simulink model "CruiseControl_TestHarness"  (R2020a)
settings: configuration reference "ModelReferencingVisual" (kept outside this file)
libraries: SignalEditorBlockLib x1
settings Model: DataDictionary=CruiseControl_Req_dd.sldd  Creator=colosky  LastModifiedBy=promero
settings ConfigSetRef: SourceName=ModelReferencingVisual

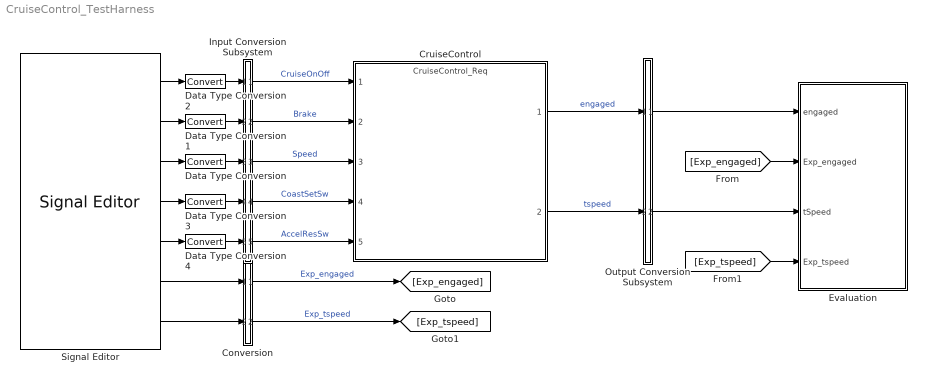
== system CruiseControl_TestHarness ==
  Conversion : Subsystem
      mask Display: disp('');
  CruiseControl : ModelReference  ModelNameDialog=CruiseControl_Req  SimulationMode=Normal  CodeInterface=Top model  ModelReferenceVersion=1.469
  Data Type Conversion{,1..4} (5 alike) : DataTypeConversion
  Evaluation : Subsystem
  Input Conversion Subsystem : Subsystem  Tag=__SLT_ICS__  Description=|
      | Signal spec.
      | and routing
      settings: AttributesFormatString=%<Description>
  Output Conversion Subsystem : Subsystem  Tag=__SLT_OCS__  Description=|
      | Signal spec.
      | and routing
      settings: AttributesFormatString=%<Description>
  Signal Editor : SignalEditorBlockLib/Signal Editor  FileName=TestInputs.mat  ActiveScenario=Engage_AccelResSw_Veh_Spd  ActiveSignal=Speed  IsBus=off  OutputBusObjectStr=Bus: BusObject  SampleTime=0.1  OutputAfterFinalValue=Extrapolation  Unit=inherit  PreserveSignalName=on
  wires:
  Conversion/1(Out6) -> [Exp_engaged]  "Exp_engaged"
  Conversion/2(Out7) -> [Exp_tspeed]  "Exp_tspeed"
  Output Conversion Subsystem/1(Outport_1) -> Evaluation/1(engaged)
  Output Conversion Subsystem/2(Outport_2) -> Evaluation/3(tSpeed)
  [Exp_engaged] -> Evaluation/2(Exp_engaged)
  [Exp_tspeed] -> Evaluation/4(Exp_tspeed)
  CruiseControl/1 -> Output Conversion Subsystem/1(Inport_1)  "engaged"
  CruiseControl/2 -> Output Conversion Subsystem/2(Inport_2)  "tspeed"
  Input Conversion Subsystem/1(Outport_1) -> CruiseControl/1  "CruiseOnOff"
  Input Conversion Subsystem/2(Outport_2) -> CruiseControl/2  "Brake"
  Input Conversion Subsystem/3(Outport_3) -> CruiseControl/3  "Speed"
  Input Conversion Subsystem/4(Outport_4) -> CruiseControl/4  "CoastSetSw"
  Input Conversion Subsystem/5(Outport_5) -> CruiseControl/5  "AccelResSw"
  Signal Editor/7 -> Conversion/2(In7)
  Signal Editor/1 -> Data Type Conversion2/1
  Signal Editor/3 -> Data Type Conversion/1
  Signal Editor/5 -> Data Type Conversion4/1
  Signal Editor/4 -> Data Type Conversion3/1
  Signal Editor/2 -> Data Type Conversion1/1
  Signal Editor/6 -> Conversion/1(In6)
  Data Type Conversion2/1 -> Input Conversion Subsystem/1(Inport_1)
  Data Type Conversion1/1 -> Input Conversion Subsystem/2(Inport_2)
  Data Type Conversion/1 -> Input Conversion Subsystem/3(Inport_3)
  Data Type Conversion3/1 -> Input Conversion Subsystem/4(Inport_4)
  Data Type Conversion4/1 -> Input Conversion Subsystem/5(Inport_5)

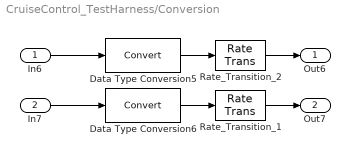
== system CruiseControl_TestHarness/Conversion ==
  In6 : Inport
  In7 : Inport  Port=2
  Data Type Conversion5 : DataTypeConversion
  Data Type Conversion6 : DataTypeConversion
  Rate_Transition_1 : RateTransition  OutPortSampleTime=0.1
  Rate_Transition_2 : RateTransition  OutPortSampleTime=0.1
  Out6 : Outport  VectorParamsAs1DForOutWhenUnconnected=off
  Out7 : Outport  Port=2  VectorParamsAs1DForOutWhenUnconnected=off
  wires:
  Data Type Conversion5/1 -> Rate_Transition_2/1
  In6/1 -> Data Type Conversion5/1
  Data Type Conversion6/1 -> Rate_Transition_1/1
  In7/1 -> Data Type Conversion6/1
  Rate_Transition_2/1 -> Out6/1
  Rate_Transition_1/1 -> Out7/1

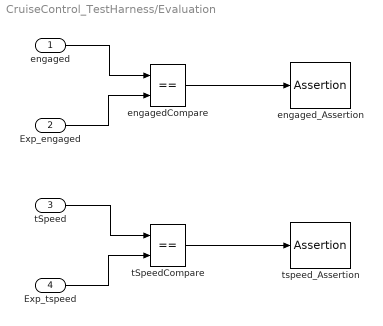
== system CruiseControl_TestHarness/Evaluation ==
  engaged : Inport
  Exp_engaged : Inport  Port=2
  tSpeed : Inport  Port=3
  Exp_tspeed : Inport  Port=4
  engagedCompare : RelationalOperator  Operator===  OutDataTypeStr=boolean  RndMeth=Nearest  InputSameDT=on
  engaged_Assertion : Assertion  StopWhenAssertionFail=off
  tSpeedCompare : RelationalOperator  Operator===  OutDataTypeStr=boolean  RndMeth=Nearest  InputSameDT=on
  tspeed_Assertion : Assertion  StopWhenAssertionFail=off
  wires:
  Exp_engaged/1 -> engagedCompare/2
  engaged/1 -> engagedCompare/1
  Exp_tspeed/1 -> tSpeedCompare/2
  tSpeed/1 -> tSpeedCompare/1
  engagedCompare/1 -> engaged_Assertion/1
  tSpeedCompare/1 -> tspeed_Assertion/1

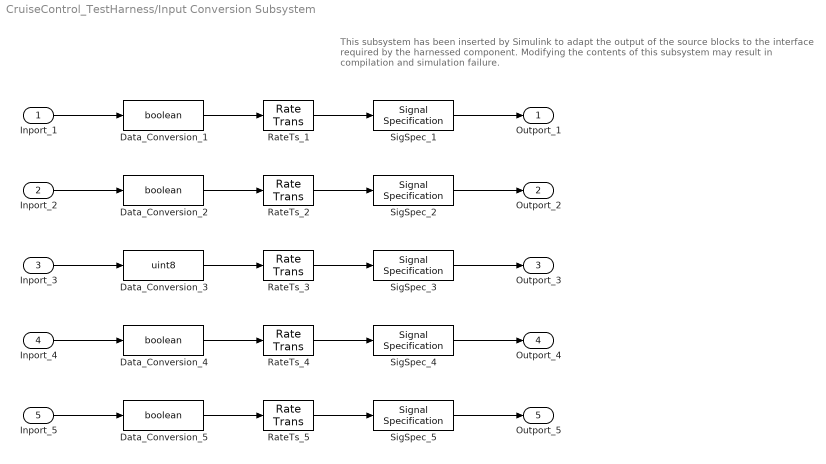
== system CruiseControl_TestHarness/Input Conversion Subsystem ==
  note: This subsystem has been inserted by Simulink to adapt the output of the source blocks to the interface required by the harnessed component.
      |  Modifying the contents of this subsystem may result in compilation and simulation failure.
  Inport_1 : Inport
  Inport_2 : Inport  Port=2
  Inport_3 : Inport  Port=3
  Inport_4 : Inport  Port=4
  Inport_5 : Inport  Port=5
  Data_Conversion_{1..2,4..5} (4 alike) : DataTypeConversion  OutDataTypeStr=boolean  SaturateOnIntegerOverflow=on  RndMeth=Zero
  Data_Conversion_3 : DataTypeConversion  OutDataTypeStr=uint8  SaturateOnIntegerOverflow=on  RndMeth=Zero
  RateTs_{1..5} (5 alike) : RateTransition  OutPortSampleTime=0.1
  SigSpec_{1..2,4..5} (4 alike) : SignalSpecification  OutDataTypeStr=boolean  Dimensions=[1]  SampleTime=0.1
  SigSpec_3 : SignalSpecification  OutDataTypeStr=uint8  Dimensions=[1]  SampleTime=0.1
  Outport_1 : Outport
  Outport_2 : Outport  Port=2
  Outport_3 : Outport  Port=3
  Outport_4 : Outport  Port=4
  Outport_5 : Outport  Port=5
  wires:
  SigSpec_1/1 -> Outport_1/1
  RateTs_1/1 -> SigSpec_1/1
  Data_Conversion_1/1 -> RateTs_1/1
  Inport_1/1 -> Data_Conversion_1/1
  SigSpec_2/1 -> Outport_2/1
  RateTs_2/1 -> SigSpec_2/1
  Data_Conversion_2/1 -> RateTs_2/1
  Inport_2/1 -> Data_Conversion_2/1
  SigSpec_3/1 -> Outport_3/1
  RateTs_3/1 -> SigSpec_3/1
  Data_Conversion_3/1 -> RateTs_3/1
  Inport_3/1 -> Data_Conversion_3/1
  SigSpec_4/1 -> Outport_4/1
  RateTs_4/1 -> SigSpec_4/1
  Data_Conversion_4/1 -> RateTs_4/1
  Inport_4/1 -> Data_Conversion_4/1
  SigSpec_5/1 -> Outport_5/1
  RateTs_5/1 -> SigSpec_5/1
  Data_Conversion_5/1 -> RateTs_5/1
  Inport_5/1 -> Data_Conversion_5/1

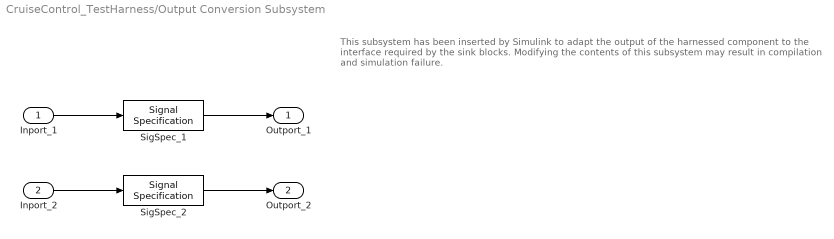
== system CruiseControl_TestHarness/Output Conversion Subsystem ==
  note: This subsystem has been inserted by Simulink to adapt the output of the harnessed component to the interface required by the sink blocks.
      |  Modifying the contents of this subsystem may result in compilation and simulation failure.
  Inport_1 : Inport
  Inport_2 : Inport  Port=2
  SigSpec_1 : SignalSpecification  OutDataTypeStr=boolean  Dimensions=[1]  SampleTime=0.1
  SigSpec_2 : SignalSpecification  OutDataTypeStr=uint8  Dimensions=[1]  SampleTime=0.1
  Outport_1 : Outport
  Outport_2 : Outport  Port=2
  wires:
  Inport_1/1 -> SigSpec_1/1
  SigSpec_1/1 -> Outport_1/1
  Inport_2/1 -> SigSpec_2/1
  SigSpec_2/1 -> Outport_2/1
